simulink model "NineLevelNEW"  (R2017a)
settings: Solver=VariableStepAuto  StartTime=0.0  StopTime=1  FixedStep=1e-5  MaxStep=1e-4  RelTol=1e-3
libraries: powerlib x22, simulink x4
settings Model: Creator=acer  LastModifiedBy=acer

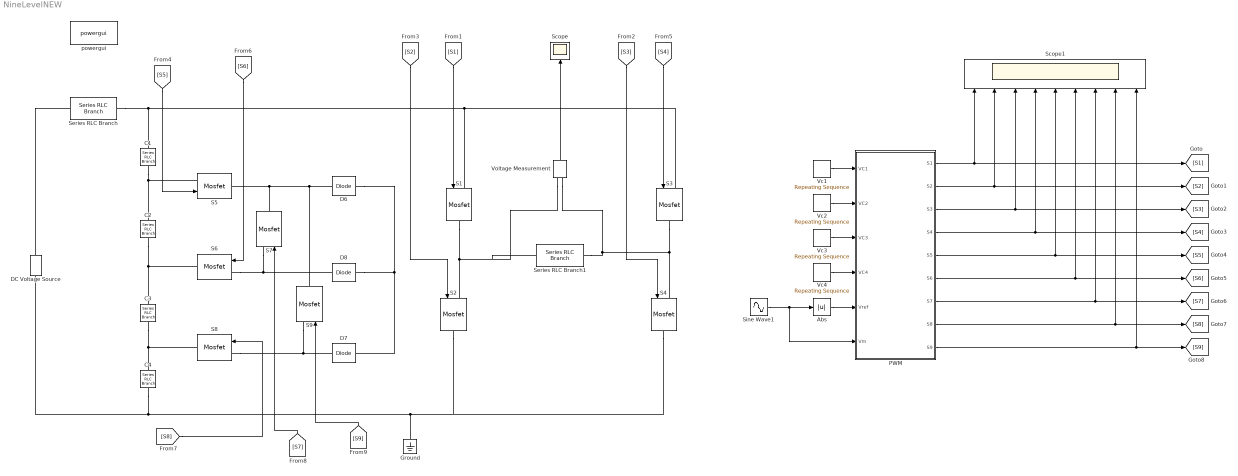
== system NineLevelNEW ==
  Abs : Abs
  C{1..4} (4 alike) : powerlib/Elements/Series RLC Branch  LConnTagsString=__new0  RConnTagsString=__new0  BranchType=C  Resistance=100  Inductance=1e-3  SetiL0=off  InitialCurrent=0  Capacitance=2  Setx0=off  InitialVoltage=0  Measurements=None
  D6 : powerlib/Power Electronics/Diode  Ron=0.001  Lon=0  Vf=.05  IC=0  UseSnubber=off  Rs=500  Cs=250e-9  Measurements=off
  D7 : powerlib/Power Electronics/Diode  Ron=0.001  Lon=0  Vf=.05  IC=0  UseSnubber=off  Rs=500  Cs=250e-9  Measurements=off
  D8 : powerlib/Power Electronics/Diode  Ron=0.001  Lon=0  Vf=.05  IC=0  UseSnubber=off  Rs=500  Cs=250e-9  Measurements=off
  DC Voltage Source : powerlib/Electrical Sources/DC Voltage Source  Amplitude=20  Measurements=None
  Ground : powerlib/Elements/Ground  LConnTagsString=a
  PWM : Subsystem
  S{1..9} (9 alike) : powerlib/Power Electronics/Mosfet  Ron=0.1  Lon=0  Rd=0.01  Vfd=0  IC=0  Rs=1e5  Cs=inf  Measurements=off
  Scope : Scope
  Scope1 : Scope  NumInputPorts=9
  Series RLC Branch : powerlib/Elements/Series RLC Branch  LConnTagsString=__new0  RConnTagsString=__new0  BranchType=R  Resistance=1e-10  Inductance=1e-3  SetiL0=off  InitialCurrent=0  Capacitance=1e-6  Setx0=off  InitialVoltage=0  Measurements=None
  Series RLC Branch1 : powerlib/Elements/Series RLC Branch  LConnTagsString=__new0  RConnTagsString=__new0  BranchType=R  Resistance=20  Inductance=1e-3  SetiL0=off  InitialCurrent=0  Capacitance=1e-6  Setx0=off  InitialVoltage=0  Measurements=None
  Sine Wave1 : Sin  Amplitude=4  Frequency=2*pi*50  SampleTime=0  VectorParams1D=off
  Vc1 : simulink/Sources/Repeating Sequence  rep_seq_t="[0  1e-4 2e-4]"  rep_seq_y=[0 1 0]
  Vc2 : simulink/Sources/Repeating Sequence  rep_seq_t="[0  1e-4 2e-4]"  rep_seq_y=[1 2 1]
  Vc3 : simulink/Sources/Repeating Sequence  rep_seq_t="[0  1e-4 2e-4]"  rep_seq_y=[2 3 2]
  Vc4 : simulink/Sources/Repeating Sequence  rep_seq_t="[0  1e-4 2e-4]"  rep_seq_y=[3 4 3]
  Voltage Measurement : powerlib/Measurements/Voltage Measurement  PhasorSimulation=off  OutputType=Complex  PSBequivalent=0
  powergui : powerlib/powergui  Priority=1  SimulationMode=Continuous  SampleTime=50e-6  frequency=60  Iterations=50  frequencyindice=0  Pbase=100e6  ErrMax=1e-4  UnitsV=kV  UnitsW=MW  buscounter=0  FunctionMessages=off  echomessages=off  EnableUseOfTLC=off  CurrentSourceSwitches=off  DisableSnubberDevices=off  DisableRonSwitches=off  DisableVfSwitches=off  DisplayEquations=off  SolverType=Tustin/Backward Euler (TBE)  Interpol=off  ExternalGateDelay=off  methode=off  Ts=100  x0status=blocks  SPID=on  SwTol=0  HookPort=off  RestoreLinks=warning  ResistiveCurrentMeasurement=off  Frange=[0:2:500]  Ylog=off  Xlog=on  ShowGrid=off  save=off  variable=ZData  structure=0  ZoomFFT=off  StartTime=0.0  cycles=1  DisplayStyle=1  fundamental=60  FreqAxis=off  MaxFrequency=1000  frequencyindicesteady=1  RmsSteady=1  display=off
  wires:
  [S4] -> S3/1
  [S3] -> S4/1
  [S1] -> S1/1
  [S2] -> S2/1
  [S5] -> S5/1
  [S6] -> S6/1
  [S8] -> S8/1
  [S7] -> S7/1
  [S9] -> S9/1
  PWM/8(S8) -> Scope1/8, [S8]
  PWM/9(S9) -> Scope1/9, [S9]
  PWM/2(S2) -> Scope1/2, [S2]
  PWM/5(S5) -> Scope1/5, [S5]
  PWM/4(S4) -> Scope1/4, [S4]
  Vc4/1 -> PWM/4(VC4)
  Vc3/1 -> PWM/3(VC3)
  Vc2/1 -> PWM/2(VC2)
  Sine Wave1/1 -> PWM/6(Vm), Abs/1
  PWM/3(S3) -> Scope1/3, [S3]
  Abs/1 -> PWM/5(Vref)
  PWM/7(S7) -> Scope1/7, [S7]
  Vc1/1 -> PWM/1(VC1)
  PWM/1(S1) -> Scope1/1, [S1]
  PWM/6(S6) -> Scope1/6, [S6]
  Voltage Measurement/1 -> Scope/1
  connections:
  Series RLC Branch/RConn1 -- C1/LConn1 -- S1/LConn1 -- S3/LConn1
  Series RLC Branch1/RConn1 -- Voltage Measurement/LConn2 -- S4/LConn1 -- S3/RConn1
  S2/RConn1 -- S4/RConn1 -- C4/RConn1 -- DC Voltage Source/LConn1 -- Ground/LConn1
  S1/RConn1 -- Voltage Measurement/LConn1 -- Series RLC Branch1/LConn1 -- S2/LConn1
  Series RLC Branch/LConn1 -- DC Voltage Source/RConn1
  C1/RConn1 -- S5/LConn1 -- C2/LConn1
  C2/RConn1 -- S6/RConn1 -- C3/LConn1
  C3/RConn1 -- S8/RConn1 -- C4/LConn1
  D6/LConn1 -- S9/RConn1 -- S7/RConn1 -- S5/RConn1
  S8/LConn1 -- S9/LConn1 -- D7/RConn1
  D6/RConn1 -- D8/LConn1 -- D7/LConn1
  S6/LConn1 -- S7/LConn1 -- D8/RConn1

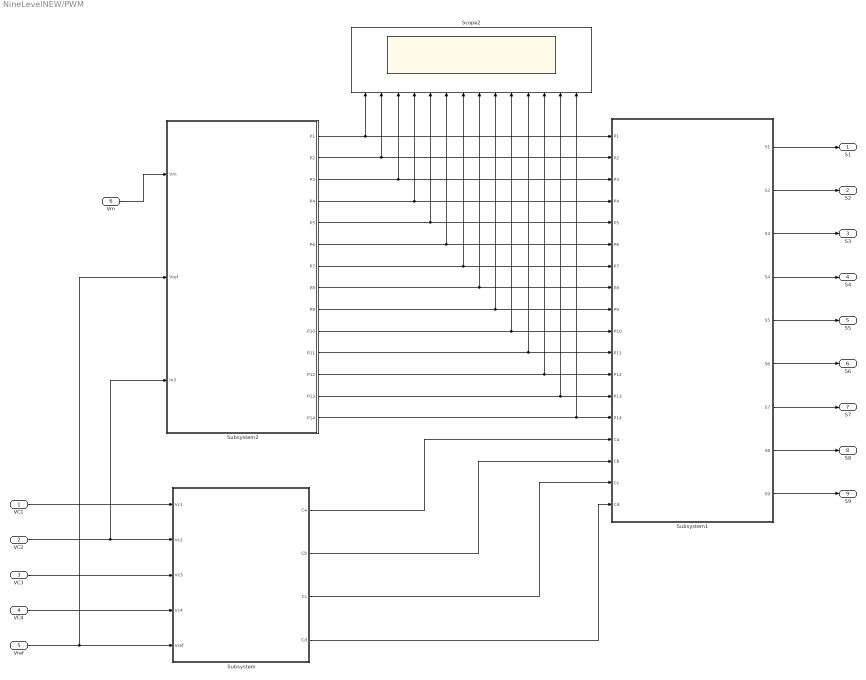
== system NineLevelNEW/PWM ==
  VC1 : Inport
  VC2 : Inport  Port=2
  VC3 : Inport  Port=3
  VC4 : Inport  Port=4
  Vref : Inport  Port=5
  Vm : Inport  Port=6
  Scope2 : Scope  NumInputPorts=14
  Subsystem : Subsystem
  Subsystem1 : Subsystem
  Subsystem2 : Subsystem
  S1 : Outport
  S2 : Outport  Port=2
  S3 : Outport  Port=3
  S4 : Outport  Port=4
  S5 : Outport  Port=5
  S6 : Outport  Port=6
  S7 : Outport  Port=7
  S8 : Outport  Port=8
  S9 : Outport  Port=9
  wires:
  Subsystem/1(Ca) -> Subsystem1/15(Ca)
  Subsystem/3(Cc) -> Subsystem1/17(Cc)
  Subsystem1/1(S1) -> S1/1
  Subsystem1/6(S6) -> S6/1
  Subsystem1/2(S2) -> S2/1
  VC1/1 -> Subsystem/1(Vc1)
  VC3/1 -> Subsystem/3(Vc3)
  Subsystem1/9(S9) -> S9/1
  Subsystem/4(Cd) -> Subsystem1/18(Cd)
  VC4/1 -> Subsystem/4(Vc4)
  Subsystem1/5(S5) -> S5/1
  Subsystem1/3(S3) -> S3/1
  VC2/1 -> Subsystem2/3(In3), Subsystem/2(Vc2)
  Subsystem1/4(S4) -> S4/1
  Subsystem/2(Cb) -> Subsystem1/16(Cb)
  Subsystem1/8(S8) -> S8/1
  Subsystem1/7(S7) -> S7/1
  Subsystem2/14(P14) -> Scope2/14, Subsystem1/14(P14)
  Subsystem2/12(P12) -> Scope2/12, Subsystem1/12(P12)
  Subsystem2/8(P8) -> Scope2/8, Subsystem1/8(P8)
  Subsystem2/7(P7) -> Scope2/7, Subsystem1/7(P7)
  Subsystem2/2(P2) -> Scope2/2, Subsystem1/2(P2)
  Subsystem2/6(P6) -> Scope2/6, Subsystem1/6(P6)
  Subsystem2/11(P11) -> Scope2/11, Subsystem1/11(P11)
  Subsystem2/1(P1) -> Scope2/1, Subsystem1/1(P1)
  Subsystem2/10(P10) -> Scope2/10, Subsystem1/10(P10)
  Subsystem2/4(P4) -> Scope2/4, Subsystem1/4(P4)
  Subsystem2/3(P3) -> Scope2/3, Subsystem1/3(P3)
  Subsystem2/9(P9) -> Scope2/9, Subsystem1/9(P9)
  Subsystem2/13(P13) -> Scope2/13, Subsystem1/13(P13)
  Subsystem2/5(P5) -> Scope2/5, Subsystem1/5(P5)
  Vm/1 -> Subsystem2/1(Vm)
  Vref/1 -> Subsystem2/2(Vref), Subsystem/5("Vref ")

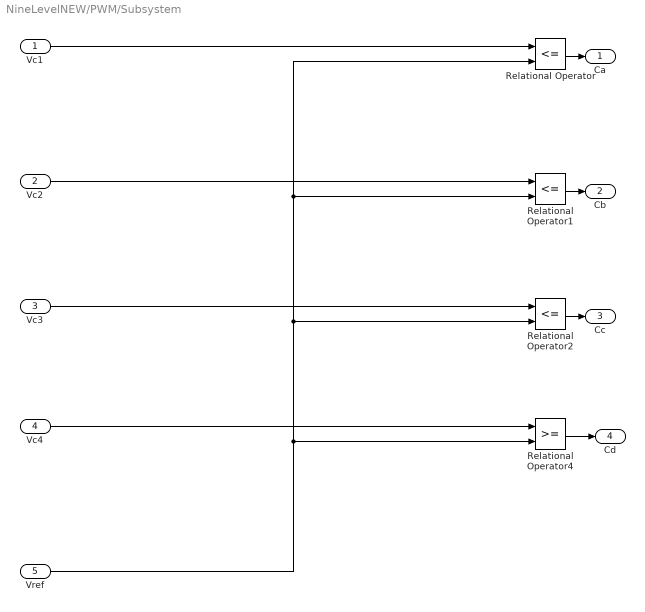
== system NineLevelNEW/PWM/Subsystem ==
  Vc1 : Inport
  Vc2 : Inport  Port=2
  Vc3 : Inport  Port=3
  Vc4 : Inport  Port=4
  "Vref " : Inport  Port=5
  Relational Operator : RelationalOperator  Operator=<=  OutDataTypeStr=boolean  RndMeth=Simplest
  Relational Operator1 : RelationalOperator  Operator=<=  OutDataTypeStr=boolean  RndMeth=Simplest
  Relational Operator2 : RelationalOperator  Operator=<=  OutDataTypeStr=boolean  RndMeth=Simplest
  Relational Operator4 : RelationalOperator  OutDataTypeStr=boolean  RndMeth=Simplest
  Ca : Outport
  Cb : Outport  Port=2
  Cc : Outport  Port=3
  Cd : Outport  Port=4
  wires:
  Vc2/1 -> Relational Operator1/1
  Vc3/1 -> Relational Operator2/1
  Relational Operator/1 -> Ca/1
  Relational Operator2/1 -> Cc/1
  Relational Operator1/1 -> Cb/1
  Vc1/1 -> Relational Operator/1
  "Vref "/1 -> Relational Operator4/2, Relational Operator2/2, Relational Operator/2, Relational Operator1/2
  Relational Operator4/1 -> Cd/1
  Vc4/1 -> Relational Operator4/1

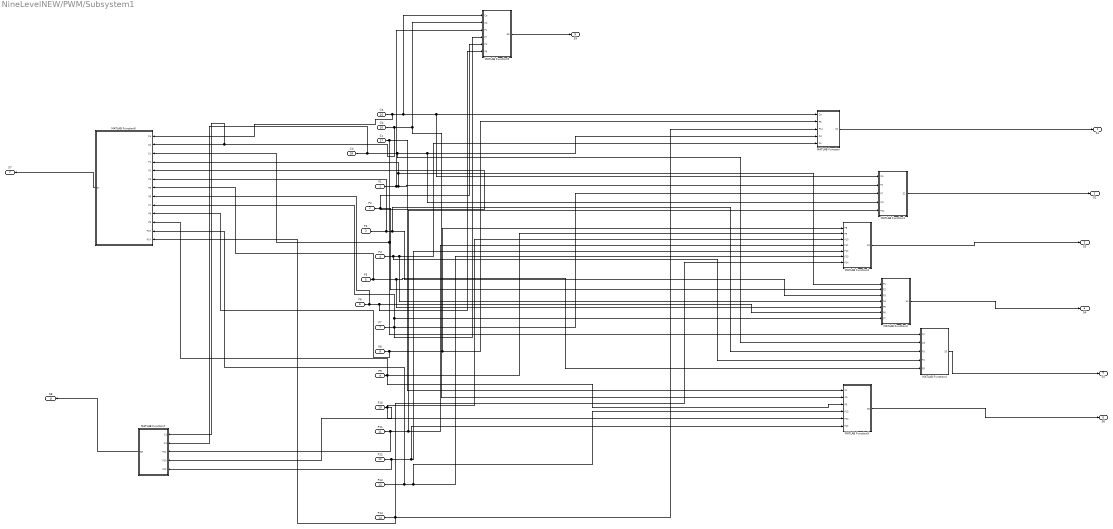
== system NineLevelNEW/PWM/Subsystem1 ==
  P1 : Inport
  P2 : Inport  Port=2
  P3 : Inport  Port=3
  P4 : Inport  Port=4
  P5 : Inport  Port=5
  P6 : Inport  Port=6
  P7 : Inport  Port=7
  P8 : Inport  Port=8
  P9 : Inport  Port=9
  P10 : Inport  Port=10
  P11 : Inport  Port=11
  P12 : Inport  Port=12
  P13 : Inport  Port=13
  P14 : Inport  Port=14
  Ca : Inport  Port=15
  Cb : Inport  Port=16
  Cc : Inport  Port=17
  Cd : Inport  Port=18
  MATLAB Function : MATLAB Function  TreatAsAtomicUnit=on
  MATLAB Function1 : MATLAB Function  TreatAsAtomicUnit=on
  MATLAB Function2 : MATLAB Function  TreatAsAtomicUnit=on
  MATLAB Function3 : MATLAB Function  TreatAsAtomicUnit=on
  MATLAB Function4 : MATLAB Function  TreatAsAtomicUnit=on
  MATLAB Function5 : MATLAB Function  TreatAsAtomicUnit=on
  MATLAB Function6 : MATLAB Function  TreatAsAtomicUnit=on
  MATLAB Function7 : MATLAB Function  TreatAsAtomicUnit=on
  MATLAB Function9 : MATLAB Function  TreatAsAtomicUnit=on
  S1 : Outport
  S2 : Outport  Port=2
  S3 : Outport  Port=3
  S4 : Outport  Port=4
  S5 : Outport  Port=5
  S6 : Outport  Port=6
  S7 : Outport  Port=7
  S8 : Outport  Port=8
  S9 : Outport  Port=9
  wires:
  Cd/1 -> MATLAB Function7/2(Cd), MATLAB Function4/2(Cd), MATLAB Function1/4(Cd), MATLAB Function/4(Cd)
  P8/1 -> MATLAB Function6/10(P8), MATLAB Function2/1(P8), MATLAB Function/2(P8)
  P4/1 -> MATLAB Function4/4(P4), MATLAB Function3/4(P4), MATLAB Function/5(P4)
  P14/1 -> MATLAB Function6/13(P14), MATLAB Function2/7(P14), MATLAB Function/3(P14)
  MATLAB Function/1(S1) -> S1/1
  P1/1 -> MATLAB Function9/3(P1), MATLAB Function6/4(P1), MATLAB Function3/1(P1), MATLAB Function1/2(P1)
  P11/1 -> MATLAB Function7/3(P11), MATLAB Function2/4(P11), MATLAB Function1/5(P11)
  MATLAB Function1/1(S2) -> S2/1
  P9/1 -> MATLAB Function6/11(P9), MATLAB Function5/3(P9), MATLAB Function2/2(P9)
  P10/1 -> MATLAB Function7/4(P10), MATLAB Function2/3(P10), MATLAB Function5/5(P10)
  P12/1 -> MATLAB Function7/5(P12), MATLAB Function5/6(P12), MATLAB Function2/5(P12)
  P13/1 -> MATLAB Function6/12(P13), MATLAB Function5/4(P13), MATLAB Function2/6(P13)
  MATLAB Function2/1(S3) -> S3/1
  MATLAB Function3/1(S4) -> S4/1
  P7/1 -> MATLAB Function9/4(P7), MATLAB Function6/9(P7), MATLAB Function3/7(P7), MATLAB Function1/3(P7)
  P6/1 -> MATLAB Function6/8(P6), MATLAB Function9/6(P6), MATLAB Function3/6(P6)
  P5/1 -> MATLAB Function6/7(P5), MATLAB Function4/5(P5), MATLAB Function3/5(P5)
  P3/1 -> MATLAB Function6/6(P3), MATLAB Function4/3(P3), MATLAB Function3/3(P3)
  P2/1 -> MATLAB Function9/5(P2), MATLAB Function6/5(P2), MATLAB Function3/2(P2)
  MATLAB Function4/1(S5) -> S5/1
  Cc/1 -> MATLAB Function5/1(Cc), MATLAB Function4/1(Cc), MATLAB Function6/3(Cc)
  MATLAB Function5/1(S6) -> S6/1
  Cb/1 -> MATLAB Function7/1(Cc), MATLAB Function6/2(Cb), MATLAB Function9/2(Cb), MATLAB Function5/2(Cb)
  MATLAB Function6/1(S7) -> S7/1
  MATLAB Function7/1(S8) -> S8/1
  MATLAB Function9/1(S9) -> S9/1
  Ca/1 -> MATLAB Function6/1(Ca), MATLAB Function9/1(Ca), MATLAB Function1/1(Ca), MATLAB Function/1(Ca)

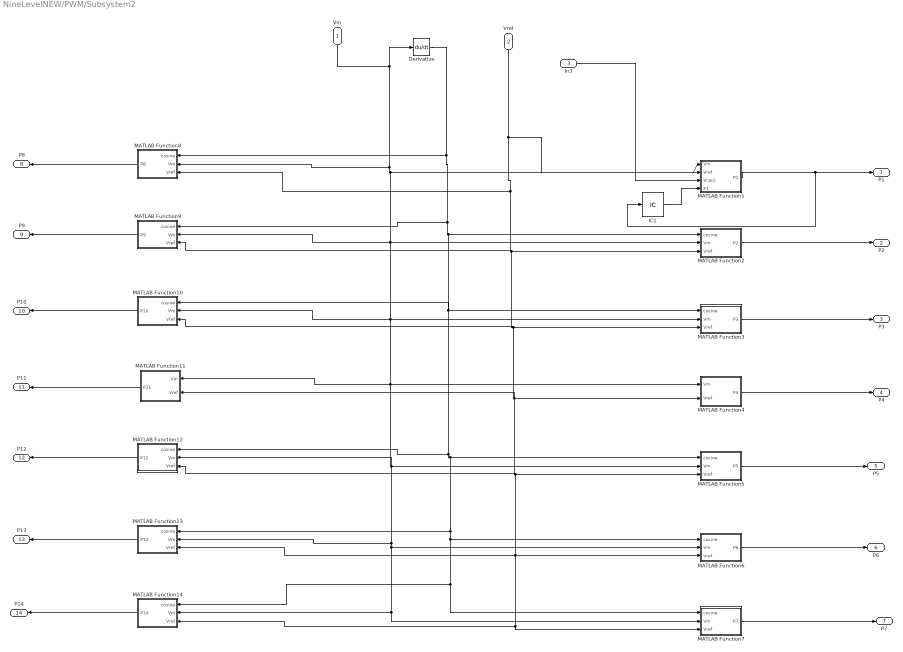
== system NineLevelNEW/PWM/Subsystem2 ==
  Vm : Inport
  Vref : Inport  Port=2
  In3 : Inport  Port=3
  Derivative : Derivative
  IC1 : InitialCondition  Value=0
  MATLAB Function1 : MATLAB Function  TreatAsAtomicUnit=on
  MATLAB Function10 : MATLAB Function  TreatAsAtomicUnit=on
  MATLAB Function11 : MATLAB Function  TreatAsAtomicUnit=on
  MATLAB Function12 : MATLAB Function  TreatAsAtomicUnit=on
  MATLAB Function13 : MATLAB Function  TreatAsAtomicUnit=on
  MATLAB Function14 : MATLAB Function  TreatAsAtomicUnit=on
  MATLAB Function2 : MATLAB Function  TreatAsAtomicUnit=on
  MATLAB Function3 : MATLAB Function  TreatAsAtomicUnit=on
  MATLAB Function4 : MATLAB Function  TreatAsAtomicUnit=on
  MATLAB Function5 : MATLAB Function  TreatAsAtomicUnit=on
  MATLAB Function6 : MATLAB Function  TreatAsAtomicUnit=on
  MATLAB Function7 : MATLAB Function  TreatAsAtomicUnit=on
  MATLAB Function8 : MATLAB Function  TreatAsAtomicUnit=on
  MATLAB Function9 : MATLAB Function  TreatAsAtomicUnit=on
  P1 : Outport
  P2 : Outport  Port=2
  P3 : Outport  Port=3
  P4 : Outport  Port=4
  P5 : Outport  Port=5
  P6 : Outport  Port=6
  P7 : Outport  Port=7
  P8 : Outport  Port=8
  P9 : Outport  Port=9
  P10 : Outport  Port=10
  P11 : Outport  Port=11
  P12 : Outport  Port=12
  P13 : Outport  Port=13
  P14 : Outport  Port=14
  wires:
  Vm/1 -> Derivative/1, MATLAB Function8/2(Vm), MATLAB Function9/2(Vm), MATLAB Function10/2(Vm), MATLAB Function11/1(Vm), MATLAB Function12/2(Vm), MATLAB Function13/2(Vm), MATLAB Function6/2(Vm), MATLAB Function14/2(Vm), MATLAB Function7/2(Vm), MATLAB Function5/2(Vm), MATLAB Function4/1(Vm), MATLAB Function3/2(Vm), MATLAB Function2/2(Vm), MATLAB Function1/1(Vm)
  MATLAB Function1/1(P1) -> IC1/1, P1/1
  MATLAB Function2/1(P2) -> P2/1
  MATLAB Function3/1(P3) -> P3/1
  MATLAB Function4/1(P4) -> P4/1
  MATLAB Function5/1(P5) -> P5/1
  MATLAB Function6/1(P6) -> P6/1
  MATLAB Function7/1(P7) -> P7/1
  MATLAB Function8/1(P8) -> P8/1
  MATLAB Function9/1(P9) -> P9/1
  MATLAB Function10/1(P10) -> P10/1
  MATLAB Function11/1(P11) -> P11/1
  MATLAB Function12/1(P12) -> P12/1
  MATLAB Function13/1(P13) -> P13/1
  MATLAB Function14/1(P14) -> P14/1
  Derivative/1 -> MATLAB Function8/1(cosine), MATLAB Function9/1(cosine), MATLAB Function10/1(cosine), MATLAB Function12/1(cosine), MATLAB Function13/1(cosine), MATLAB Function6/1(cosine), MATLAB Function14/1(cosine), MATLAB Function7/1(cosine), MATLAB Function5/1(cosine), MATLAB Function3/1(cosine), MATLAB Function2/1(cosine)
  Vref/1 -> MATLAB Function1/2(Vref), MATLAB Function8/3(Vref), MATLAB Function9/3(Vref), MATLAB Function10/3(Vref), MATLAB Function11/2(Vref), MATLAB Function12/3(Vref), MATLAB Function13/3(Vref), MATLAB Function6/3(Vref), MATLAB Function14/3(Vref), MATLAB Function7/3(Vref), MATLAB Function5/3(Vref), MATLAB Function4/2(Vref), MATLAB Function3/3(Vref), MATLAB Function2/3(Vref)
  In3/1 -> MATLAB Function1/3(Vcar2)
  IC1/1 -> MATLAB Function1/4("P1 ")

== matlab function NineLevelNEW/PWM/Subsystem1/MATLAB Function ==
  data: Ca input; S1 output; P8 input; P14 input; Cd input; P4 input
function S1 = fcn(Ca,P8,P14,Cd,P4)
S1 = ((Ca&&(P8||P14))||(Cd&&P4));

== matlab function NineLevelNEW/PWM/Subsystem1/MATLAB Function1 ==
  data: Ca input; S2 output; P1 input; P7 input; Cd input; P11 input
function S2 = fcn(Ca,P1,P7,Cd,P11)
S2 = (Ca&&(P1||P7))||(Cd&&P11);

== matlab function NineLevelNEW/PWM/Subsystem1/MATLAB Function2 ==
  data: P8 input; S3 output; P9 input; P10 input; P11 input; P12 input; P13 input; P14 input
function S3 = fcn(P8,P9,P10,P11,P12,P13,P14)
S3 = (P8||P9||P10||P11||P12||P13||P14);

== matlab function NineLevelNEW/PWM/Subsystem1/MATLAB Function3 ==
  data: P1 input; S4 output; P2 input; P3 input; P4 input; P5 input; P6 input; P7 input
function S4 = fcn(P1,P2, P3,P4,P5,P6,P7)
S4 = (P1||P2||P3||P4||P5||P6||P7);

== matlab function NineLevelNEW/PWM/Subsystem1/MATLAB Function4 ==
  data: Cc input; S5 output; Cd input; P3 input; P4 input; P5 input
function S5 = fcn(Cc,Cd, P3,P4,P5)
S5 = (Cc&&(P3||P5))||(Cd&&P4);

== matlab function NineLevelNEW/PWM/Subsystem1/MATLAB Function5 ==
  data: Cc input; S6 output; Cb input; P9 input; P13 input; P10 input; P12 input
function S6 = fcn(Cc,Cb, P9,P13,P10,P12)
S6 = (Cb&&(P9||P13))||(Cc&&(P10||P12));

== matlab function NineLevelNEW/PWM/Subsystem1/MATLAB Function6 ==
  data: Ca input; Cb input; Cc input; P1 input; P2 input; P3 input; P5 input; P6 input; P7 input; P8 input; S7 output; P9 input; P13 input; P14 input
function S7 = fcn(Ca,Cb,Cc,P1,P2, P3,P5,P6,P7,P8,P9,P13,P14)
S7 = (Ca && (P8||P14)) || (Cc && (P3||P5)) || (Cb && (P9||P13)) || (Cb && (P1||P2||P6||P7));

== matlab function NineLevelNEW/PWM/Subsystem1/MATLAB Function7 ==
  data: Cc input; S8 output; Cd input; P11 input; P10 input; P12 input
function S8 = fcn(Cc,Cd,P11,P10,P12)
S8 = (Cc&&(P10||P12))||(Cd&&P11);

== matlab function NineLevelNEW/PWM/Subsystem2/MATLAB Function1 ==
  data: Vm input; Vref input; P1 output; Vcar2 input; P1 input
function P1 = fcn( Vm, Vref, Vcar2, P1)
while(Vm>0)
    if (Vref == Vcar2)
        break;
    end
    P1 = 1;
end

== matlab function NineLevelNEW/PWM/Subsystem1/MATLAB Function9 ==
  data: Ca input; S9 output; Cb input; P1 input; P7 input; P2 input; P6 input
function S9 = fcn(Ca,Cb, P1,P7,P2,P6)
S9 = (Ca&&(P1||P7))||(Cb &&(P2||P6));

== matlab function NineLevelNEW/PWM/Subsystem2/MATLAB Function2 ==
  data: cosine input; Vm input; P2 output; Vref input
function P2 = fcn(cosine, Vm, Vref)
if (Vm>=0) && (cosine>=0) && (Vref>=1) &&(Vref <= 2)
    P2=1;
else
    P2 = 0;
end

== matlab function NineLevelNEW/PWM/Subsystem2/MATLAB Function3 ==
  data: cosine input; Vm input; P3 output; Vref input
function P3 = fcn(cosine, Vm, Vref)
if (Vm>=0) && (cosine>=0) && (Vref>=2) &&(Vref <= 3)
    P3=1;
else
    P3 = 0;
end

== matlab function NineLevelNEW/PWM/Subsystem2/MATLAB Function4 ==
  data: Vm input; P4 output; Vref input
function P4 = fcn(   Vm, Vref)
if (Vm>=0) &&  (Vref>=3) &&(Vref <= 4)
    P4=1;
else
    P4 = 0;
end

== matlab function NineLevelNEW/PWM/Subsystem2/MATLAB Function5 ==
  data: cosine input; Vm input; P5 output; Vref input
function P5 = fcn(cosine, Vm, Vref)
if (Vm>=0) && (cosine<=0) && (Vref>=2) &&(Vref <= 3)
    P5=1;
else
    P5 = 0;
end

== matlab function NineLevelNEW/PWM/Subsystem2/MATLAB Function6 ==
  data: cosine input; Vm input; P6 output; Vref input
function P6 = fcn(cosine, Vm, Vref)
if (Vm>=0) && (cosine<=0) && (Vref>=1) &&(Vref <= 2)
    P6=1;
else
    P6 = 0;
end

== matlab function NineLevelNEW/PWM/Subsystem2/MATLAB Function7 ==
  data: cosine input; Vm input; P7 output; Vref input
function P7 = fcn(cosine, Vm, Vref)
if (Vm>=0) && (cosine<=0) && (Vref>=0) &&(Vref <= 1)
    P7=1;
else
    P7 = 0;
end

== matlab function NineLevelNEW/PWM/Subsystem2/MATLAB Function10 ==
  data: cosine input; Vm input; P10 output; Vref input
function P10 = fcn(cosine, Vm, Vref)
if (Vm<=0) && (cosine<=0) && (Vref>=2) &&(Vref <= 3)
    P10=1;
else
    P10= 0;
end

== matlab function NineLevelNEW/PWM/Subsystem2/MATLAB Function11 ==
  data: Vm input; P11 output; Vref input
function P11 = fcn(   Vm, Vref)
if (Vm<=0) &&  (Vref>=3) &&(Vref <= 4)
    P11=1;
else
    P11 = 0;
end

== matlab function NineLevelNEW/PWM/Subsystem2/MATLAB Function12 ==
  data: cosine input; Vm input; P12 output; Vref input
function P12 = fcn(cosine, Vm, Vref)
if (Vm<0) && (cosine>=0) && (Vref>=2) &&(Vref <= 3)
    P12=1;
else
    P12 = 0;
end

== matlab function NineLevelNEW/PWM/Subsystem2/MATLAB Function13 ==
  data: cosine input; Vm input; P13 output; Vref input
function P13 = fcn(cosine, Vm, Vref)
if (Vm<0) && (cosine>=0) && (Vref>=1) &&(Vref <= 2)
    P13=1;
else
    P13 = 0;
end

== matlab function NineLevelNEW/PWM/Subsystem2/MATLAB Function14 ==
  data: cosine input; Vm input; P14 output; Vref input
function P14 = fcn(cosine, Vm, Vref)
if (Vm<0) && (cosine>=0) && (Vref>=0) &&(Vref <= 1)
    P14=1;
else
    P14 = 0;
end

== matlab function NineLevelNEW/PWM/Subsystem2/MATLAB Function8 ==
  data: cosine input; Vm input; P8 output; Vref input
function P8 = fcn(cosine, Vm, Vref)
if (Vm<=0) && (cosine<=0) && (Vref>=0) &&(Vref <= 1)
    P8=1;
else
    P8 = 0;
end

== matlab function NineLevelNEW/PWM/Subsystem2/MATLAB Function9 ==
  data: cosine input; Vm input; P9 output; Vref input
function P9 = fcn(cosine, Vm, Vref)
if (Vm<=0) && (cosine<=0) && (Vref>=1) &&(Vref <= 2)
    P9=1;
else
    P9 = 0;
end
